simulink model "ring_modulator"  (R2017a)
settings: Solver=VariableStepAuto  StartTime=0.0  StopTime=inf  RelTol=1e-3
libraries: dspvision x1, dspsrcs4 x1, dspobslib x1
settings Model: Creator=ilyas  LastModifiedBy=ilyas

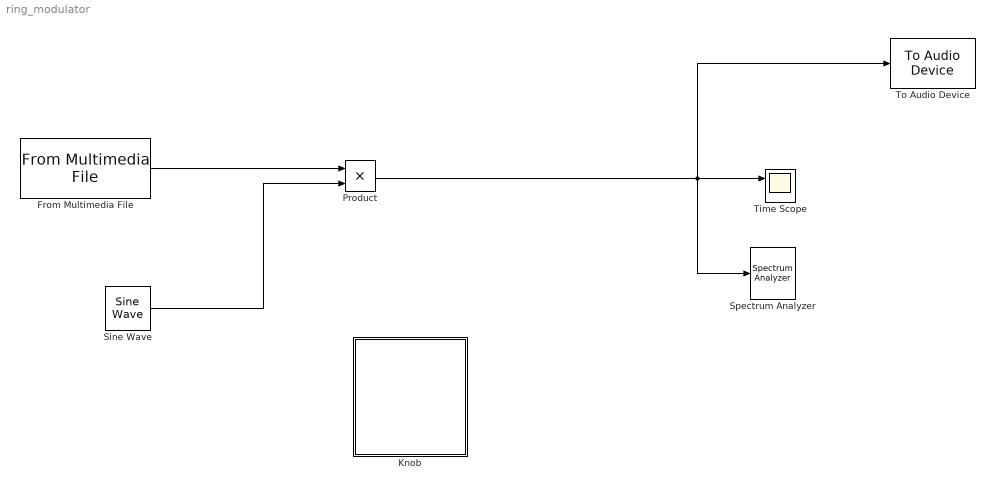
== system ring_modulator ==
  From Multimedia File : dspvision/From Multimedia File  inputFilename=C:\Users\ilyas\Desktop\cours UPMC\Son et image\audio\tpaudio\guitare.wav  loop=on  numPlays=inf  outputStreams=Audio only  videoDataType=single  audioDataType=double  inheritSampleTime=on  userDefinedSampleTime=1/30  noAudioOutput=off  isIntensityVideo=off  fourcc=RGB  colorVideoFormat=Separate color signals  outputEOF=off  dataOrg=Column-major  audioFrameSize=1024  computeAudioFrameSize=off  outSamplingMode=Sample based
      settings: SourceProductBaseCode=VP
  Knob : Subsystem  DialogController=hmiCreateDDGDialog  IsWebBlock=on  mask(MWDashboardBlock){webBlockId=7d11c1b0-9d79-421c-bd63-6e862e6bd707, webBlockType=continuousknob, ShowInLibBrowser=on, ShowInitialText=on, HMISrcModelName=ring_modulator}
      mask prompts: webBlockId "WebBlock Id"; webBlockType "WebBlock Type"; HMISrcModelName "Source Model"
      mask help: SimulinkHMI:dialogs:ContinuousKnobDialogDesc
      mask Help: helpview([docroot '/mapfiles/simulink.map'], 'hmi_knob')
      mask Display:
      | if strcmp(get_param(bdroot(gcb),'BlockDiagramType'), 'library')
      |     image([(matlabroot) '/toolbox/simulink/hmi/icons/ContinuousKnob.png']);
      | end
  Product : Product
  Sine Wave : dspsrcs4/Sine Wave  Amplitude=1  Frequency=659.23806975683  Phase=0  SampleMode=Discrete  OutComplex=Real  CompMethod=Trigonometric fcn  TableSize=Speed  SampleTime=1/11025  SamplesPerFrame=1024  ResetState=Restart at time zero  OutputFrames=off  dataType=double  wordLen=16  udDataType=sfix(16)  fracBitsMode=Best precision  numFracBits=15  OutDataTypeStr=double  LastOutDataTypeStr=double
  Spectrum Analyzer : SpectrumAnalyzer
  Time Scope : Scope  NumInputPorts=2
  To Audio Device : dspobslib/To Audio Device  deviceName=Default  inheritSampleRate=on  sampleRate=44100  deviceDatatype=Determine from input data type  autoBufferSize=on  bufferSize=4096  queueDuration=1.0  defaultOutputChannelMapping=on  outputChannelMapping=1:2  outputNumUnderrunSamples=off
      settings: SourceProductName=DSP System Toolbox  SourceProductBaseCode=DS
  wires:
  Sine Wave/1 -> Product/2
  Product/1 -> To Audio Device/1, Spectrum Analyzer/1, Time Scope/1
  From Multimedia File/1 -> Product/1

== system ring_modulator/Knob ==
